simulink model "closedloop_estimator"  (R2015a)
settings: Solver=ode45  StartTime=0.0  StopTime=10  FixedStep=1e-3  MaxStep=1e-2  RelTol=1e-3
undefined symbols (not defined in the file): A, B, C, L
settings Model: Creator=henrik  LastModifiedBy=hg35a
settings DataIOCC: SignalLoggingSaveFormat=ModelDataLogs  SignalLoggingName=sigsOut
settings OptimizationCC: ExpressionDepthLimit=2147483647  InitFltsAndDblsToZero=on
settings DebuggingCC: SaveWithParameterizedLinksMsg=none  UnderspecifiedInitializationDetection=Classic  MergeDetectMultiDrivingBlocksExec=none  SignalResolutionControl=TryResolveAllWithWarning  MultiTaskDSMMsg=warning  MultiTaskCondExecSysMsg=none  FcnCallInpInsideContextMsg=UseLocalSettings  StateNameClashWarn=warning
settings HardwareCC: TargetUnknown=on
settings GRTTargetCC: TargetFcnLib=ansi_tfl_tmw.mat  ModelReferenceCompliant=off  CombineOutputUpdateFcns=off  MatFileLogging=off  GRTInterface=on

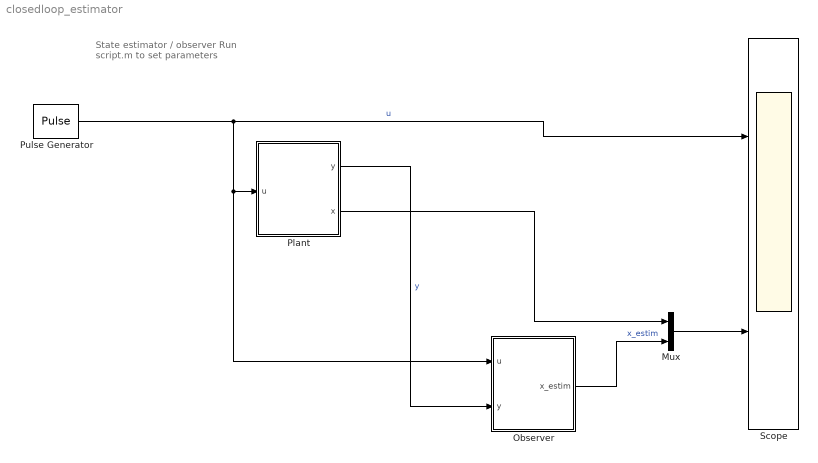
== system closedloop_estimator ==
  note: State estimator / observer
      | Run script.m to set parameters
  Mux : Mux  Inputs=2
  Observer : Subsystem
  Plant : Subsystem
  Pulse Generator : DiscretePulseGenerator  PulseType=Time based  Amplitude=10*pi/180  Period=10  PulseWidth=50
      settings: AttributesFormatString=Amplitude=%<Amplitude>
  Scope : Scope  NumInputPorts=2
      settings: YMin=-1~0  YMax=1.5~0.02
  wires:
  Pulse Generator/1 -> Observer/1(u), Plant/1(u), Scope/1  "u"
  Plant/1(y) -> Observer/2(y)  "y"
  Plant/2(x) -> Mux/1
  Observer/1(x_estim) -> Mux/2  "x_estim"
  Mux/1 -> Scope/2

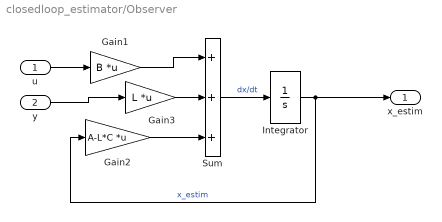
== system closedloop_estimator/Observer ==
  u : Inport
  y : Inport  Port=2
  Gain1 : Gain  Gain=B  Multiplication=Matrix(K*u)  SaturateOnIntegerOverflow=on  OutDataTypeStr=Inherit: Same as input  ParamDataTypeStr=Inherit: Same as input
  Gain2 : Gain  Gain=A-L*C  Multiplication=Matrix(K*u)  SaturateOnIntegerOverflow=on  OutDataTypeStr=Inherit: Same as input  ParamDataTypeStr=Inherit: Same as input
  Gain3 : Gain  Gain=L  Multiplication=Matrix(K*u)  SaturateOnIntegerOverflow=on  OutDataTypeStr=Inherit: Same as input  ParamDataTypeStr=Inherit: Same as input
  Integrator : Integrator
  Sum : Sum  Inputs=+++  SaturateOnIntegerOverflow=on  InputSameDT=on  OutDataTypeStr=Inherit: Same as first input
  x_estim : Outport
  wires:
  u/1 -> Gain1/1
  Sum/1 -> Integrator/1  "dx/dt"
  Integrator/1 -> Gain2/1, x_estim/1  "x_estim"
  Gain1/1 -> Sum/1
  Gain2/1 -> Sum/3
  y/1 -> Gain3/1
  Gain3/1 -> Sum/2

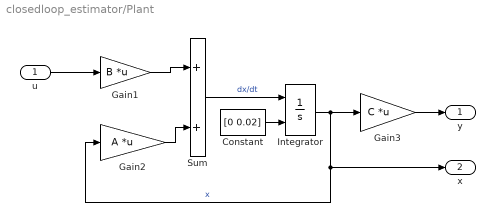
== system closedloop_estimator/Plant ==
  u : Inport
  Constant : Constant  Value=[0 0.02]
  Gain1 : Gain  Gain=B  Multiplication=Matrix(K*u)  SaturateOnIntegerOverflow=on  OutDataTypeStr=Inherit: Same as input  ParamDataTypeStr=Inherit: Same as input
  Gain2 : Gain  Gain=A  Multiplication=Matrix(K*u)  SaturateOnIntegerOverflow=on  OutDataTypeStr=Inherit: Same as input  ParamDataTypeStr=Inherit: Same as input
  Gain3 : Gain  Gain=C  Multiplication=Matrix(K*u)  SaturateOnIntegerOverflow=on  OutDataTypeStr=Inherit: Same as input  ParamDataTypeStr=Inherit: Same as input
  Integrator : Integrator  InitialConditionSource=external
  Sum : Sum  SaturateOnIntegerOverflow=on  InputSameDT=on  OutDataTypeStr=Inherit: Same as first input
  y : Outport
  x : Outport  Port=2
  wires:
  Gain1/1 -> Sum/1
  Constant/1 -> Integrator/2
  Gain2/1 -> Sum/2
  Integrator/1 -> Gain3/1, Gain2/1, x/1  "x"
  Sum/1 -> Integrator/1  "dx/dt"
  Gain3/1 -> y/1
  u/1 -> Gain1/1
